simulink model "ParkTransform"  (R2022a)
settings: Solver=VariableStepAuto  StartTime=0.0  StopTime=10.0  RelTol=1e-3
settings Model: Creator=jff_1  LastModifiedBy=jff_1

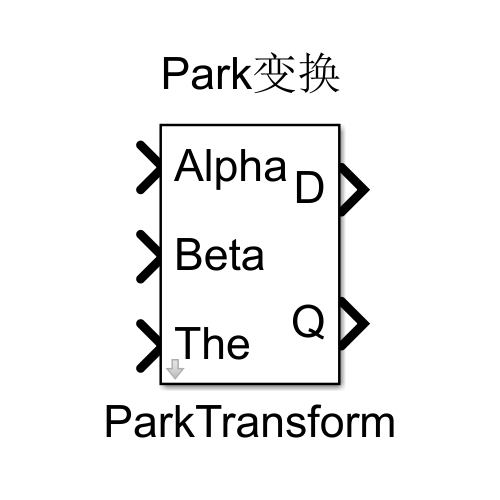
[thumbnail: Simulink's stored preview of the top-level diagram]
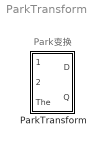
== system ParkTransform ==
  note: Park变换
  ParkTransform : Subsystem
      mask help:
      | Park 变换用于将静止 α-β 坐标系中的物理量转换到同步旋转 d-q 坐标系。
      |
      | 通过引入同步旋转角 θ（通常为电角度），将 α-β 平面上的矢量
      | 旋转到以转子磁场为参考的 d-q 坐标系中，使交流量在稳态下
      | 转化为直流量，便于控制器设计与分析。
      |
      | 该变换广泛应用于永磁同步电机（PMSM）和异步电机的矢量控制中，
      | 是磁场定向控制（FOC）的核心坐标变换之一。
      mask Help:
      | 【功能说明】
      | 本模块实现 Park 坐标变换，将 α-β 静止坐标系下的输入量
      | 转换为同步旋转坐标系下的 d-q 分量。
      | 
      | 【数学表达式】
      | 设输入为：
      |   α  —— α 轴分量
      |   β  —— β 轴分量
      |   θ  —— 同步旋转角（电角度，单位：rad）
      | 
      | 则 Park 变换公式为：
      | 
      |   d =  α·cos(θ) + β·sin(θ)
      |   q = -α·sin(θ) + β·cos(θ)
      | 
      | 矩阵形式表示为：
      | 
      |   [ d ] = [  cosθ   sinθ ] [ α ]
      |   [ q ]   [ -sinθ   cosθ ] [ β ]
      | 
      | 【端口说明】
      | 输入端口：
      |   α     —— α 轴分量
      |   β     —— β 轴分量
      |   θ     —— 同步旋转角（rad）
      | 
      | 输出端口：
      |   d     —— d 轴分量
      |   q     —— q 轴分量
      | 
      | 【使用说明】
      | 1. θ 通常由转子位置或积分电角速度获得；
      | 2. 在 PMSM 矢量控制中：
      |    - d 轴通常用于磁链控制
      |    - q 轴通常用于转矩控制
      | 3. 若 α-β 来自 Clarke 变换，则该模块构成完整的
      |    abc → αβ → dq 坐标变换链路。
      | 
      | 【注意事项】
      | - 本模块未包含零序分量；
      | - 输入信号应满足单位一致性（θ 为弧度制）。
      mask DialogControl ParameterGroupVar Prompt: 参数
      mask Display:
      | % 输入端口标签（1~3）
      | port_label('input',1,'Alpha');
      | port_label('input',2,'Beta');
      | port_label('input',3,'The');
      | 
      | % 输出端口标签（1~2）
      | port_label('output',1,'D');
      | port_label('output',2,'Q');

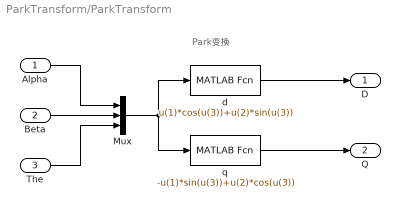
== system ParkTransform/ParkTransform ==
  note: Park变换
  Alpha : Inport
  Beta : Inport  Port=2
  The : Inport  Port=3
  Mux : Mux  Inputs=3
  d : MATLABFcn  MATLABFcn=u(1)*cos(u(3))+u(2)*sin(u(3))
  q : MATLABFcn  MATLABFcn=-u(1)*sin(u(3))+u(2)*cos(u(3))
  D : Outport
  Q : Outport  Port=2
  wires:
  d/1 -> D/1
  The/1 -> Mux/3
  Mux/1 -> q/1, d/1
  q/1 -> Q/1
  Alpha/1 -> Mux/1
  Beta/1 -> Mux/2
